simulink model "StateSpace"  (R2014b)
settings: Solver=ode45  StartTime=0.0  StopTime=10.0  RelTol=1e-3
settings Model: Creator=99641  LastModifiedBy=99641

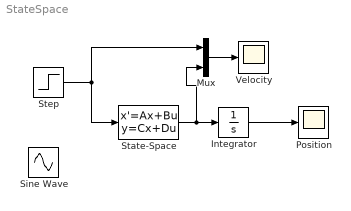
== system StateSpace ==
  Integrator : Integrator
  Mux : Mux  Inputs=2
  Position : Scope
  Sine Wave : Sin  SampleTime=0
  State-Space : StateSpace  A=[-5,-10;8,0]  B=[4;0]  C=[2.5,0]  D=0  X0=0
  Step : Step  SampleTime=0
  Velocity : Scope
  wires:
  State-Space/1 -> Mux/2, Integrator/1
  Integrator/1 -> Position/1
  Mux/1 -> Velocity/1
  Step/1 -> State-Space/1, Mux/1
